simulink model "model"  (R2023b)
settings: Solver=VariableStepAuto  StartTime=0.0  StopTime=10.0  RelTol=1e-3
undefined symbols (not defined in the file): DiscIntNeverNeededParam, fd74c4e2, magnitude, Newton, Raphson
libraries: simulink x102, slpidlib x35
(part 1 of 5)
settings Model: Creator=ojiken  LastModifiedBy=ojiken

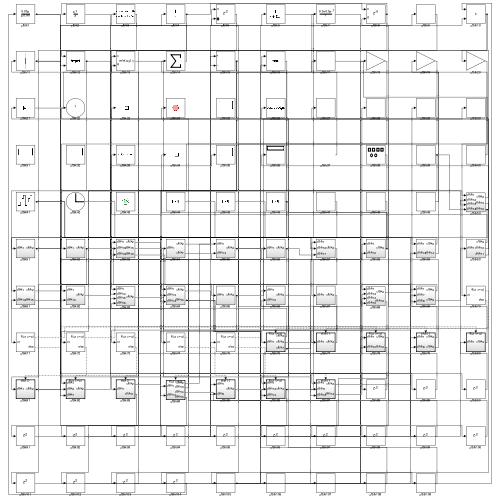
[thumbnail: Simulink's stored preview of the top-level diagram]
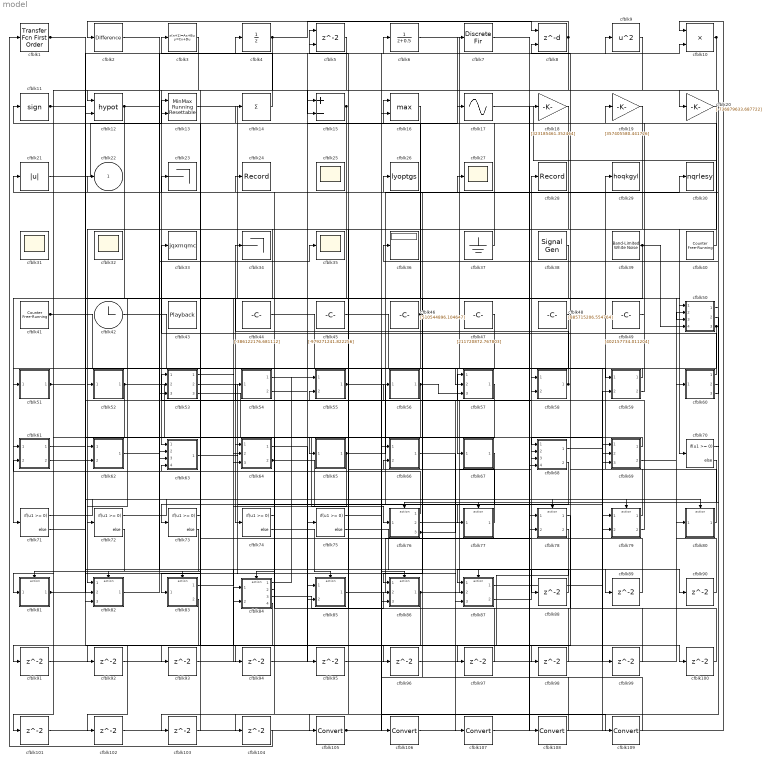
== system model ==
  cfblk1 : simulink/Discrete/Transfer Fcn First Order  PoleZ=0.95  ICPrevOutput=0.0  DoSatur=off
  cfblk10 : Product  Inputs=**
  cfblk{88..104} (17 alike) : Delay  SampleTime=1
  cfblk{105..109} (5 alike) : DataTypeConversion  SaturateOnIntegerOverflow=off  RndMeth=Floor
  cfblk11 : Signum
  cfblk12 : Math  Operator=hypot
  cfblk13 : simulink/Math Operations/MinMax Running Resettable  Function=min  vinit=0.0
  cfblk14 : Sum  Inputs=+
  cfblk15 : Sum  Inputs=+-
  cfblk16 : MinMax  Function=max  Inputs=2
  cfblk17 : Sin  TimeSource=Use external signal  SampleTime=0
  cfblk18 : Gain  Gain=[323185461.352464]
  cfblk19 : Gain  Gain=[357405580.441726]
  cfblk2 : simulink/Discrete/Difference  ICPrevInput=0.0  OutMin=[]  OutMax=[]  OutDataTypeStr=Inherit: Inherit via back propagation  OutDataType=fixdt(1, 16)  OutScaling=2^-10  DoSatur=off
  cfblk20 : Gain  Gain=[-736879633.687722]
  cfblk21 : Abs  SaturateOnIntegerOverflow=off
  cfblk23 : Terminator
  cfblk24 : Record  FileSettingsInternal="{\"entries\":[{\"content\":{\"excelSettings\":{\"content\":{},\"type\":\"Streamout.ExcelSettings\"}},\"type\":\"Streamout.FileSettingStorage\",\"uuid\":\"\"}],\"packageUris\":[\"http:\\/\\/schema.mathworks.com\\/mf0\\/streamout_blocks\\/R2020a\"],\"version\":\"1.0\"}"  SignalsInternal="{\"entries\":[{\"content\":{},\"type\":\"RecordBlkView.InputSignals\",\"uuid\":\"\"}],\"packageUris\":[\"http:\\/\\/schema.mathworks.com\\/mf0\\/streamout_blocks\\/R2020a\"],\"version\":\"1.0\"}"  VisualizationBindings="{\"sparklinesplugin\":{\"info\":[{\"bindingParametersList\":[],\"subplotID\":1}]}}"
  cfblk{25,27,31..32,35} (5 alike) : Scope
      cfblk25 settings: Floating=on
      cfblk31 settings: Floating=on
      cfblk32 settings: Floating=on
  cfblk26 : ToWorkspace  VariableName=lyoptgs  SaveFormat=Timeseries  SampleTime=-1
  cfblk28 : Record  FileSettingsInternal="{\"entries\":[{\"content\":{\"excelSettings\":{\"content\":{},\"type\":\"Streamout.ExcelSettings\"}},\"type\":\"Streamout.FileSettingStorage\",\"uuid\":\"\"}],\"packageUris\":[\"http:\\/\\/schema.mathworks.com\\/mf0\\/streamout_blocks\\/R2020a\"],\"version\":\"1.0\"}"  SignalsInternal="{\"entries\":[{\"content\":{},\"type\":\"RecordBlkView.InputSignals\",\"uuid\":\"\"}],\"packageUris\":[\"http:\\/\\/schema.mathworks.com\\/mf0\\/streamout_blocks\\/R2020a\"],\"version\":\"1.0\"}"  VisualizationBindings="{\"sparklinesplugin\":{\"info\":[{\"bindingParametersList\":[],\"subplotID\":1}]}}"
  cfblk29 : ToWorkspace  VariableName=hoqkgyl  SaveFormat=Timeseries  SampleTime=-1
  cfblk3 : DiscreteStateSpace
  cfblk30 : ToWorkspace  VariableName=nqrlesy  SaveFormat=Timeseries  SampleTime=-1
  cfblk33 : ToWorkspace  VariableName=jqxmqmc  SaveFormat=Timeseries  SampleTime=-1
  cfblk34 : Terminator
  cfblk36 : Display
  cfblk37 : Ground
  cfblk38 : SignalGenerator  Amplitude=[-773767244.573252]  Units=rad/sec
  cfblk39 : simulink/Sources/Band-Limited White Noise  Cov=[9388450366.311230]  Ts=0.1  seed=[6338139783.000000]
  cfblk4 : UnitDelay  HasFrameUpgradeWarning=on
  cfblk40 : simulink/Sources/Counter Free-Running  NumBits=[55.000000]  tsamp=-1
  cfblk41 : simulink/Sources/Counter Free-Running  NumBits=[4.000000]  tsamp=-1
  cfblk42 : Clock
  cfblk43 : Playback  NumPorts=0  PartName=fd74c4e2-0fad-4813-8d20-90b65e462531
  cfblk44 : Constant  Value=[-386122176.681112]  SampleTime=1
  cfblk45 : Constant  Value=[-979271241.822256]  SampleTime=1
  cfblk46 : Constant  Value=[510544896.104647]  SampleTime=1
  cfblk47 : Constant  Value=[211720872.767803]  SampleTime=1
  cfblk48 : Constant  Value=[885715206.554764]  SampleTime=1
  cfblk49 : Constant  Value=[402157734.011204]  SampleTime=1
  cfblk5 : Delay  ShowEnablePort=on  SampleTime=1
      settings: InputPortMap=u0,e6
  cfblk50 : Subsystem
  cfblk51 : Subsystem
  cfblk52 : Subsystem
  cfblk53 : Subsystem
  cfblk54 : Subsystem
  cfblk55 : Subsystem
  cfblk56 : Subsystem
  cfblk57 : Subsystem
  cfblk58 : Subsystem
  cfblk59 : Subsystem
  cfblk6 : DiscreteTransferFcn  SampleTime=1
  cfblk60 : Subsystem
  cfblk61 : Subsystem
  cfblk62 : Subsystem
  cfblk63 : Subsystem
  cfblk64 : Subsystem
  cfblk65 : Subsystem
  cfblk66 : Subsystem
  cfblk67 : Subsystem
  cfblk68 : Subsystem
  cfblk69 : Subsystem
  cfblk7 : DiscreteFir  SampleTime=1
  cfblk{70..75} (6 alike) : If  IfExpression=u1 >= 0  SampleTime=1
  cfblk76 : Subsystem  TreatAsAtomicUnit=on
  cfblk77 : Subsystem  TreatAsAtomicUnit=on
  cfblk78 : Subsystem  TreatAsAtomicUnit=on
  cfblk79 : Subsystem  TreatAsAtomicUnit=on
  cfblk8 : Delay  DelayLengthSource=Input port  SampleTime=1
      settings: InputPortMap=u0,p1
  cfblk80 : Subsystem  TreatAsAtomicUnit=on
  cfblk81 : Subsystem  TreatAsAtomicUnit=on
  cfblk82 : Subsystem  TreatAsAtomicUnit=on
  cfblk83 : Subsystem  TreatAsAtomicUnit=on
  cfblk84 : Subsystem  TreatAsAtomicUnit=on
  cfblk85 : Subsystem  TreatAsAtomicUnit=on
  cfblk86 : Subsystem  TreatAsAtomicUnit=on
  cfblk87 : Subsystem  TreatAsAtomicUnit=on
  cfblk9 : Math  Operator=square
  cfblk22 : Outport
  wires:
  cfblk15/1 -> cfblk72/1, cfblk64/3(cfblk14), cfblk93/1
  cfblk84/1(cfblk2) -> cfblk55/1(cfblk1)
  cfblk3/1 -> cfblk63/1(cfblk1)
  cfblk80/1(cfblk2) -> cfblk29/1
  cfblk65/1(cfblk2) -> cfblk30/1, cfblk84/2(cfblk12)
  cfblk17/1 -> cfblk70/1
  cfblk12/1 -> cfblk82/1(cfblk1), cfblk89/1
  cfblk44/1 -> cfblk76/1(cfblk1)
  cfblk39/1 -> cfblk71/1, cfblk50/4(cfblk14)
  cfblk62/1(cfblk2) -> cfblk9/1
  cfblk46/1 -> cfblk11/1, cfblk62/2(cfblk13), cfblk53/2(cfblk13)
  cfblk48/1 -> cfblk82/2(cfblk6)
  cfblk85/1(cfblk2) -> cfblk28/1
  cfblk54/1(cfblk2) -> cfblk6/1
  cfblk84/2(cfblk13) -> cfblk23/1
  cfblk47/1 -> cfblk61/1(cfblk1)
  cfblk63/1(cfblk2) -> cfblk79/2(cfblk8)
  cfblk6/1 -> cfblk59/1(cfblk1)
  cfblk8/1 -> cfblk2/1, cfblk101/1
  cfblk13/1 -> cfblk50/1(cfblk1)
  cfblk40/1 -> cfblk7/1
  cfblk41/1 -> cfblk68/4(cfblk15), cfblk106/1
  cfblk86/1(cfblk2) -> cfblk58/1(cfblk1), cfblk91/1
  cfblk49/1 -> cfblk19/1
  cfblk51/1(cfblk2) -> cfblk57/2(cfblk16), cfblk88/1
  cfblk53/2(cfblk15) -> cfblk87/2(cfblk11)
  cfblk55/1(cfblk2) -> cfblk87/3(cfblk12), cfblk10/2
  cfblk21/1 -> cfblk13/1
  cfblk45/1 -> cfblk67/1(cfblk1)
  cfblk4/1 -> cfblk83/1(cfblk1), cfblk8/1
  cfblk58/1(cfblk2) -> cfblk34/1, cfblk26/1
  cfblk69/1(cfblk2) -> cfblk68/1(cfblk1)
  cfblk82/1(cfblk2) -> cfblk35/1
  cfblk81/1(cfblk2) -> cfblk4/1, cfblk94/1
  cfblk50/1(cfblk2) -> cfblk20/1
  cfblk56/1(cfblk2) -> cfblk57/3(cfblk17), cfblk104/1
  cfblk60/1(cfblk2) -> cfblk33/1
  cfblk57/1(cfblk2) -> cfblk82/3(cfblk7)
  cfblk79/1(cfblk2) -> cfblk21/1
  cfblk14/1 -> cfblk3/1
  cfblk18/1 -> cfblk105/1
  cfblk20/1 -> cfblk52/1(cfblk1)
  cfblk37/1 -> cfblk14/1
  cfblk1/1 -> cfblk63/2(cfblk14), cfblk85/2(cfblk9)
  cfblk16/1 -> cfblk62/1(cfblk1)
  cfblk59/1(cfblk2) -> cfblk51/1(cfblk1)
  cfblk19/1 -> cfblk74/1
  cfblk5/1 -> cfblk12/1
  cfblk52/1(cfblk2) -> cfblk65/1(cfblk1), cfblk81/1(cfblk1)
  cfblk38/1 -> cfblk86/1(cfblk1)
  cfblk68/1(cfblk2) -> cfblk59/2(cfblk13)
  cfblk61/1(cfblk2) -> cfblk56/1(cfblk1)
  cfblk87/1(cfblk2) -> cfblk69/2(cfblk7)
  cfblk69/2(cfblk9) -> cfblk60/1(cfblk1)
  cfblk87/2(cfblk13) -> cfblk68/2(cfblk13)
  cfblk60/2(cfblk10) -> cfblk36/1
  cfblk9/1 -> cfblk12/2
  cfblk76/1(cfblk2) -> cfblk61/2(cfblk14)
  cfblk77/1(cfblk2) -> cfblk5/1
  cfblk10/1 -> cfblk15/2, cfblk53/3(cfblk14)
  cfblk11/1 -> cfblk5/2, cfblk50/3(cfblk13)
  cfblk60/3(cfblk11) -> cfblk22/1
  cfblk50/3(cfblk16) -> cfblk27/1, cfblk64/2(cfblk13)
  cfblk42/1 -> cfblk69/3(cfblk8)
  cfblk61/2(cfblk15) -> cfblk57/1(cfblk1)
  cfblk79/2(cfblk9) -> cfblk54/1(cfblk1)
  cfblk54/2(cfblk7) -> cfblk17/1
  cfblk64/2(cfblk15) -> cfblk53/1(cfblk1), cfblk86/3(cfblk14), cfblk100/1
  cfblk2/1 -> cfblk64/1(cfblk1)
  cfblk68/2(cfblk16) -> cfblk73/1
  cfblk76/2(cfblk6) -> cfblk68/3(cfblk14)
  cfblk67/1(cfblk2) -> cfblk77/1(cfblk1)
  cfblk59/2(cfblk14) -> cfblk16/1
  cfblk84/3(cfblk14) -> cfblk86/2(cfblk13)
  cfblk76/3(cfblk7) -> cfblk24/1, cfblk58/2(cfblk10)
  cfblk70/1 -> cfblk76/Action
  cfblk70/2 -> cfblk77/Action
  cfblk71/1 -> cfblk78/Action
  cfblk71/2 -> cfblk79/Action
  cfblk72/1 -> cfblk80/Action
  cfblk72/2 -> cfblk81/Action
  cfblk73/1 -> cfblk82/Action
  cfblk73/2 -> cfblk83/Action
  cfblk74/1 -> cfblk84/Action
  cfblk74/2 -> cfblk85/Action
  cfblk75/1 -> cfblk86/Action
  cfblk75/2 -> cfblk87/Action
  cfblk88/1 -> cfblk87/1(cfblk1)
  cfblk89/1 -> cfblk63/4(cfblk16)
  cfblk83/1(cfblk2) -> cfblk90/1
  cfblk90/1 -> cfblk50/2(cfblk12)
  cfblk91/1 -> cfblk84/1(cfblk1)
  cfblk83/2(cfblk11) -> cfblk92/1
  cfblk92/1 -> cfblk75/1
  cfblk93/1 -> cfblk79/1(cfblk1)
  cfblk94/1 -> cfblk15/1
  cfblk64/1(cfblk2) -> cfblk95/1
  cfblk95/1 -> cfblk78/1(cfblk1)
  cfblk78/1(cfblk2) -> cfblk96/1
  cfblk96/1 -> cfblk80/1(cfblk1)
  cfblk78/2(cfblk10) -> cfblk97/1
  cfblk97/1 -> cfblk85/1(cfblk1)
  cfblk53/1(cfblk2) -> cfblk98/1
  cfblk98/1 -> cfblk55/2(cfblk13)
  cfblk53/3(cfblk16) -> cfblk99/1
  cfblk99/1 -> cfblk63/3(cfblk15)
  cfblk100/1 -> cfblk8/2
  cfblk101/1 -> cfblk10/1
  cfblk84/4(cfblk15) -> cfblk102/1
  cfblk102/1 -> cfblk78/2(cfblk9)
  cfblk50/2(cfblk15) -> cfblk103/1
  cfblk103/1 -> cfblk13/2
  cfblk104/1 -> cfblk1/1
  cfblk105/1 -> cfblk16/2, cfblk109/1
  cfblk106/1 -> cfblk18/1
  cfblk66/1(cfblk2) -> cfblk107/1
  cfblk107/1 -> cfblk69/1(cfblk1)
  cfblk7/1 -> cfblk108/1
  cfblk108/1 -> cfblk66/1(cfblk1)
  cfblk109/1 -> cfblk66/2(cfblk12)

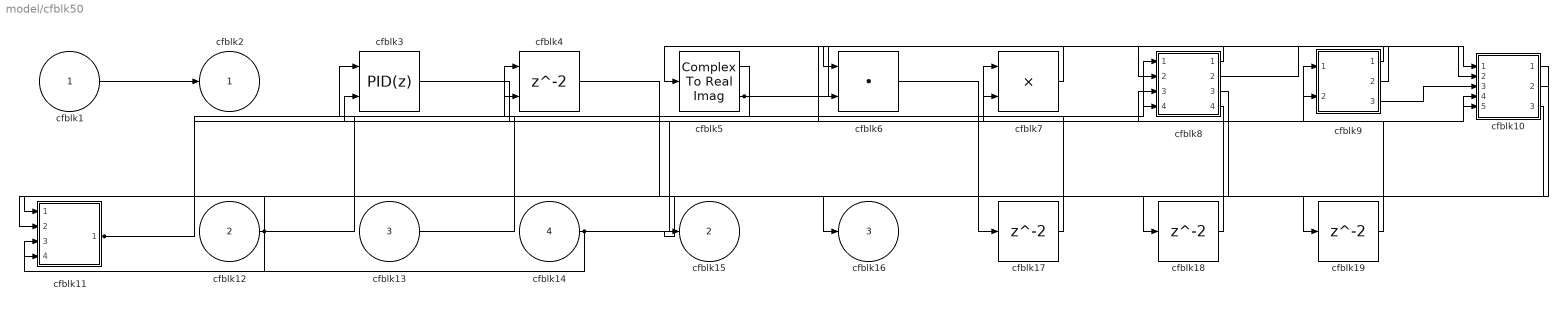
== system model/cfblk50 ==
  cfblk1 : Inport
  cfblk12 : Inport  Port=2
  cfblk13 : Inport  Port=3
  cfblk14 : Inport  Port=4
  cfblk10 : Subsystem
  cfblk11 : Subsystem
  cfblk17 : Delay  SampleTime=1
  cfblk18 : Delay  SampleTime=1
  cfblk19 : Delay  SampleTime=1
  cfblk3 : slpidlib/PID Controller (2DOF)  Controller=PID  Form=Parallel  TimeDomain=Discrete-time  UseExternalTs=off  SampleTime=1  IntegratorMethod=Forward Euler  FilterMethod=Forward Euler  ControllerParametersSource=internal  P=1  I=1  UseKiTs=off  D=0  N=100  UseFilter=on  b=1  c=1  TunerSelectOption=Transfer Function Based (PID Tuner App)  InitialConditionSource=internal  InitialConditionForIntegrator=0  InitialConditionForFilter=0  DifferentiatorICPrevScaledInput=0  ExternalReset=none  TrackingMode=off  Kt=1  LimitOutput=off  SatLimitsSource=internal  UpperSaturationLimit=inf  LowerSaturationLimit=-inf  LinearizeAsGain=off  AntiWindupMode=none  Kb=1  LimitIntegrator=off  UpperIntegratorSaturationLimit=inf  LowerIntegratorSaturationLimit=-inf  POutMin=[]  POutMax=[]  IOutMin=[]  IOutMax=[]  DOutMin=[]  DOutMax=[]  NOutMin=[]  NOutMax=[]  bOutMin=[]  bOutMax=[]  cOutMin=[]  cOutMax=[]  SumOutMin=[]  SumOutMax=[]  SaturationOutMin=[]  SaturationOutMax=[]  PParamMin=[]  PParamMax=[]  IParamMin=[]  IParamMax=[]  DParamMin=[]  DParamMax=[]  NParamMin=[]  NParamMax=[]  bParamMin=[]  bParamMax=[]  cParamMin=[]  cParamMax=[]  KbParamMin=[]  KbParamMax=[]  KtParamMin=[]  KtParamMax=[]  KbOutMin=[]  KbOutMax=[]  KtOutMin=[]  KtOutMax=[]  IntegratorOutMin=[]  IntegratorOutMax=[]  FilterOutMin=[]  FilterOutMax=[]  SumI1OutMin=[]  SumI1OutMax=[]  SumI2OutMin=[]  SumI2OutMax=[]  SumI3OutMin=[]  SumI3OutMax=[]  SumI4OutMin=[]  SumI4OutMax=[]  SumDOutMin=[]  SumDOutMax=[]  Sum1OutMin=[]  Sum1OutMax=[]  Sum2OutMin=[]  Sum2OutMax=[]  Sum3OutMin=[]  Sum3OutMax=[]  DifferentiatorOutMin=[]  DifferentiatorOutMax=[]  FilterDiffOutCoefMin=[]  FilterDiffOutCoefMax=[]  ReciprocalOutMin=[]  ReciprocalOutMax=[]  SumDenOutMin=[]  SumDenOutMax=[]  SumNumOutMin=[]  SumNumOutMax=[]  DivideOutMin=[]  DivideOutMax=[]  UdiffTsProdOutMin=[]  UdiffTsProdOutMax=[]  NTsProdOutMin=[]  NTsProdOutMax=[]  UintegralTsProdOutMin=[]  UintegralTsProdOutMax=[]  UngainTsProdOutMin=[]  UngainTsProdOutMax=[]  ClampingZeroOutDataTypeStr=Inherit: Inherit via back propagation  ClampingZeroOutMin=[]  ClampingZeroOutMax=[]  FilterDenConstantOutDataTypeStr=Inherit: Inherit via back propagation  FilterDenConstantOutMin=[]  FilterDenConstantOutMax=[]  PCopyOutDataTypeStr=Inherit: Inherit via back propagation  PCopyOutMin=[]  PCopyOutMax=[]  NCopyOutDataTypeStr=Inherit: Inherit via back propagation  NCopyOutMin=[]  NCopyOutMax=[]  IntegratorContinuousStateAttributes=''  IntegratorStateMustResolveToSignalObject=off  IntegratorRTWStateStorageClass=Auto  FilterContinuousStateAttributes=''  FilterStateMustResolveToSignalObject=off  FilterRTWStateStorageClass=Auto  ParallelPVariant=InternalParameters  IdealPVariant=Disabled  IVariant=InternalParameters  DVariant=InternalParameters  bVariant=InternalParameters  cVariant=InternalParameters  IntegratorVariant=Discrete  SatVariant=Disabled  AWVariant=Passthrough  PCopyVariant=Disabled  TRVariant=Disabled  FdbkBlocksVariant=Forward  IdealPFdbkVariant=Disabled  SatFdbkVariant=Disabled  DerivativeFilterVariant=ForwardEulerFilter  NVariant=InternalParameters  NCopyVariant=Disabled  FilterICVariant=InternalICsFilter  IntegratorICVariant=InternalICs  ExternalResetVariant=Disabled  TRSumVariant=Passthrough  SumFdbkVariant=Disabled  SumVariant=Sum_PID  TsampFilterVariant=InternalTs  TsampNgainVariant=Passthrough  TsampIntegralVariant=Disabled_SignalSpec  ExternalSaturationOutDataTypeStr=Inherit: Same as second input
      settings: LibrarySourceBlock=simulink/Discrete/Discrete PID Controller (2DOF)
  cfblk4 : Delay  ShowEnablePort=on  SampleTime=1
      settings: InputPortMap=u0,e6
  cfblk5 : ComplexToRealImag
  cfblk6 : DotProduct  OutDataTypeStr=Inherit: Inherit via internal rule
  cfblk7 : Product  Inputs=**
  cfblk8 : Subsystem
  cfblk9 : Subsystem
  cfblk2 : Outport
  cfblk15 : Outport  Port=2
  cfblk16 : Outport  Port=3
  wires:
  cfblk3/1 -> cfblk9/1(cfblk1)
  cfblk1/1 -> cfblk2/1
  cfblk12/1 -> cfblk11/1(cfblk1), cfblk7/2, cfblk8/4(cfblk11), cfblk11/4(cfblk15)
  cfblk11/1(cfblk2) -> cfblk4/1, cfblk10/4(cfblk11)
  cfblk5/1 -> cfblk4/2
  cfblk5/2 -> cfblk10/1(cfblk1), cfblk10/5(cfblk12)
  cfblk8/1(cfblk2) -> cfblk5/1
  cfblk7/1 -> cfblk6/1
  cfblk13/1 -> cfblk8/1(cfblk1)
  cfblk14/1 -> cfblk9/2(cfblk9), cfblk11/3(cfblk14)
  cfblk8/2(cfblk12) -> cfblk10/2(cfblk9)
  cfblk10/1(cfblk2) -> cfblk15/1
  cfblk9/1(cfblk2) -> cfblk6/2
  cfblk9/2(cfblk10) -> cfblk8/2(cfblk9)
  cfblk9/3(cfblk11) -> cfblk10/3(cfblk10)
  cfblk8/3(cfblk13) -> cfblk11/2(cfblk13)
  cfblk8/4(cfblk14) -> cfblk7/1
  cfblk10/2(cfblk13) -> cfblk16/1
  cfblk6/1 -> cfblk17/1
  cfblk17/1 -> cfblk3/1
  cfblk4/1 -> cfblk18/1
  cfblk18/1 -> cfblk3/2
  cfblk10/3(cfblk14) -> cfblk19/1
  cfblk19/1 -> cfblk8/3(cfblk10)

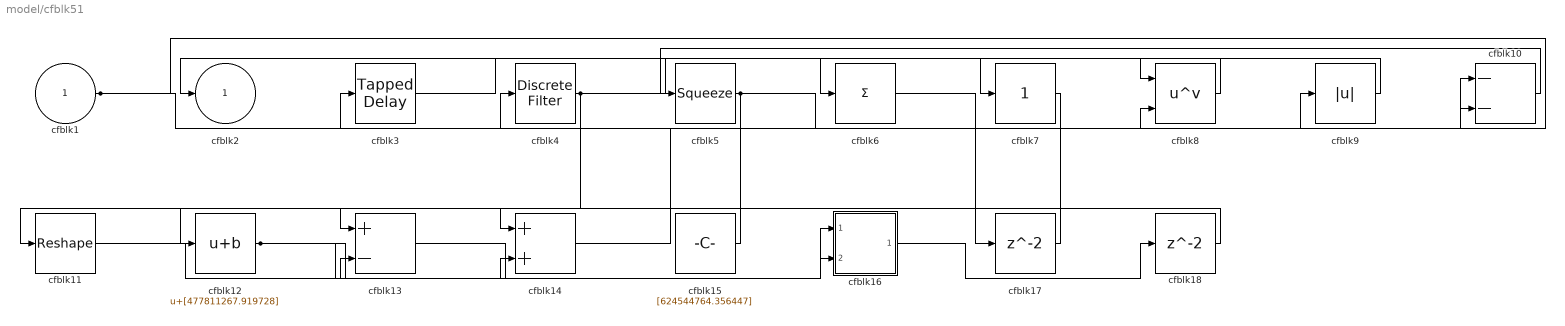
== system model/cfblk51 ==
  cfblk1 : Inport
  cfblk10 : Sum  Inputs=--
  cfblk11 : Reshape
  cfblk12 : Bias  Bias=[477811267.919728]  SaturateOnIntegerOverflow=off
  cfblk13 : Sum  Inputs=+-
  cfblk14 : Sum
  cfblk15 : Constant  Value=[624544764.356447]  SampleTime=1
  cfblk16 : Subsystem
  cfblk17 : Delay  SampleTime=1
  cfblk18 : Delay  SampleTime=1
  cfblk3 : simulink/Discrete/Tapped Delay  vinit=0.0  samptime=-1  NumDelays=1  DelayOrder=Oldest  includeCurrent=off
  cfblk4 : DiscreteFilter  SampleTime=1
  cfblk5 : Squeeze
  cfblk6 : Sum  Inputs=+
  cfblk7 : simulink/Math Operations/Slider Gain  gain=1  low=0  high=2
  cfblk8 : Math  Operator=pow
  cfblk9 : Abs  SaturateOnIntegerOverflow=off
  cfblk2 : Outport
  wires:
  cfblk7/1 -> cfblk11/1
  cfblk4/1 -> cfblk7/1, cfblk12/1
  cfblk15/1 -> cfblk4/1
  cfblk12/1 -> cfblk16/1(cfblk1), cfblk14/2
  cfblk10/1 -> cfblk5/1
  cfblk3/1 -> cfblk6/1
  cfblk11/1 -> cfblk13/2
  cfblk14/1 -> cfblk9/1
  cfblk8/1 -> cfblk2/1
  cfblk5/1 -> cfblk14/1, cfblk8/2
  cfblk9/1 -> cfblk8/1
  cfblk1/1 -> cfblk10/1, cfblk10/2
  cfblk13/1 -> cfblk16/2(cfblk11)
  cfblk6/1 -> cfblk17/1
  cfblk17/1 -> cfblk3/1
  cfblk16/1(cfblk2) -> cfblk18/1
  cfblk18/1 -> cfblk13/1

== system model/cfblk52 ==
  cfblk1 : Inport
  cfblk10 : Subsystem
  cfblk11 : Subsystem
  cfblk{12..17} (6 alike) : Delay  SampleTime=1
  cfblk3 : DiscreteStateSpace
  cfblk4 : Delay  DelayLengthSource=Input port  SampleTime=1
      settings: InputPortMap=u0,p1
  cfblk5 : Sqrt
  cfblk6 : Abs  SaturateOnIntegerOverflow=off
  cfblk7 : Subsystem
  cfblk8 : Subsystem
  cfblk9 : Subsystem
  cfblk2 : Outport
  wires:
  cfblk3/1 -> cfblk13/1, cfblk14/1
  cfblk1/1 -> cfblk8/2(cfblk6)
  cfblk7/1(cfblk2) -> cfblk9/1(cfblk1)
  cfblk5/1 -> cfblk2/1, cfblk15/1
  cfblk11/2(cfblk15) -> cfblk3/1
  cfblk7/2(cfblk12) -> cfblk10/1(cfblk1), cfblk11/2(cfblk13)
  cfblk9/1(cfblk2) -> cfblk11/1(cfblk1)
  cfblk4/1 -> cfblk7/1(cfblk1)
  cfblk11/3(cfblk16) -> cfblk5/1, cfblk16/1
  cfblk8/1(cfblk2) -> cfblk4/2, cfblk6/1
  cfblk6/1 -> cfblk10/2(cfblk6), cfblk11/3(cfblk14), cfblk10/3(cfblk7)
  cfblk11/1(cfblk2) -> cfblk12/1
  cfblk12/1 -> cfblk4/1
  cfblk13/1 -> cfblk8/1(cfblk1)
  cfblk14/1 -> cfblk9/2(cfblk7)
  cfblk15/1 -> cfblk8/3(cfblk7)
  cfblk16/1 -> cfblk8/4(cfblk8)
  cfblk10/1(cfblk2) -> cfblk17/1
  cfblk17/1 -> cfblk7/2(cfblk11)

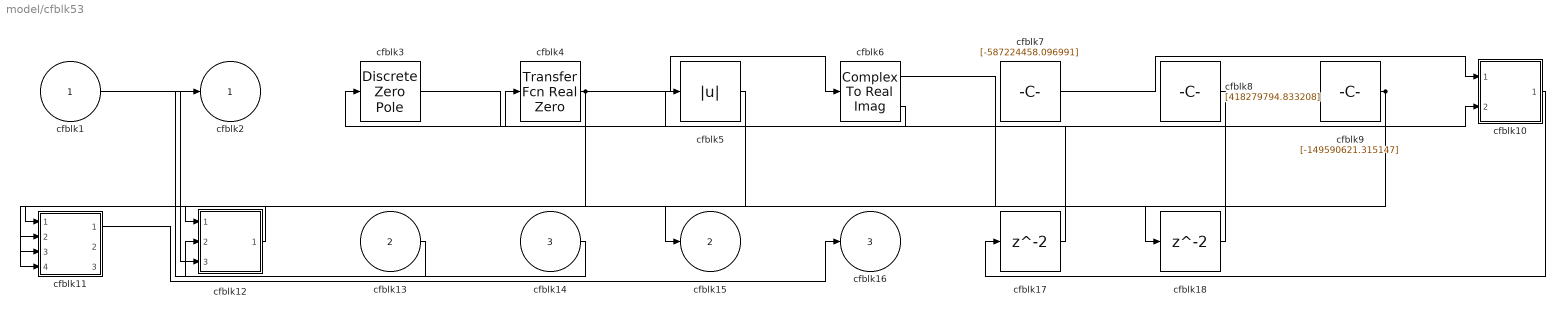
== system model/cfblk53 ==
  cfblk1 : Inport
  cfblk13 : Inport  Port=2
  cfblk14 : Inport  Port=3
  cfblk10 : Subsystem
  cfblk11 : Subsystem
  cfblk12 : Subsystem
  cfblk17 : Delay  SampleTime=1
  cfblk18 : Delay  SampleTime=1
  cfblk3 : DiscreteZeroPole  Poles=[0 0.5]  Gain=1
  cfblk4 : simulink/Discrete/Transfer Fcn Real Zero  ZeroZ=0.75  ICPrevInput=0.0  DoSatur=off
  cfblk5 : Abs  SaturateOnIntegerOverflow=off
  cfblk6 : ComplexToRealImag
  cfblk7 : Constant  Value=[-587224458.096991]  SampleTime=1
  cfblk8 : Constant  Value=[418279794.833208]  SampleTime=1
  cfblk9 : Constant  Value=[-149590621.315147]  SampleTime=1
  cfblk2 : Outport
  cfblk15 : Outport  Port=2
  cfblk16 : Outport  Port=3
  wires:
  cfblk9/1 -> cfblk12/1(cfblk1), cfblk11/3(cfblk8)
  cfblk14/1 -> cfblk2/1
  cfblk7/1 -> cfblk10/1(cfblk1)
  cfblk4/1 -> cfblk6/1, cfblk11/4(cfblk9)
  cfblk6/2 -> cfblk5/1
  cfblk8/1 -> cfblk15/1
  cfblk11/1(cfblk2) -> cfblk16/1
  cfblk3/1 -> cfblk10/2(cfblk10)
  cfblk13/1 -> cfblk12/2(cfblk13)
  cfblk1/1 -> cfblk12/3(cfblk14)
  cfblk12/1(cfblk2) -> cfblk11/1(cfblk1)
  cfblk5/1 -> cfblk11/2(cfblk7)
  cfblk10/1(cfblk2) -> cfblk17/1
  cfblk17/1 -> cfblk3/1
  cfblk6/1 -> cfblk18/1
  cfblk18/1 -> cfblk4/1

== system model/cfblk54 ==
  cfblk1 : Inport
  cfblk{4,8..10} (4 alike) : Delay  SampleTime=1
  cfblk3 : Delay  DelayLengthSource=Input port  SampleTime=1
      settings: InputPortMap=u0,p1
  cfblk5 : MinMax  Inputs=3
  cfblk6 : Gain  Gain=[-108671966.700826]
  cfblk2 : Outport
  cfblk7 : Outport  Port=2
  wires:
  cfblk1/1 -> cfblk2/1
  cfblk6/1 -> cfblk8/1, cfblk9/1
  cfblk5/1 -> cfblk6/1
  cfblk4/1 -> cfblk7/1, cfblk5/2, cfblk10/1
  cfblk3/1 -> cfblk4/1, cfblk5/3
  cfblk8/1 -> cfblk5/1
  cfblk9/1 -> cfblk3/1
  cfblk10/1 -> cfblk3/2

== system model/cfblk55 ==
  cfblk1 : Inport
  cfblk13 : Inport  Port=2
  cfblk10 : Subsystem
  cfblk11 : Subsystem
  cfblk12 : Subsystem
  cfblk{14..17} (4 alike) : Delay  SampleTime=1
  cfblk3 : slpidlib/PID Controller (2DOF)  Controller=PID  Form=Parallel  TimeDomain=Discrete-time  UseExternalTs=off  SampleTime=1  IntegratorMethod=Forward Euler  FilterMethod=Forward Euler  ControllerParametersSource=internal  P=1  I=1  UseKiTs=off  D=0  N=100  UseFilter=on  b=1  c=1  TunerSelectOption=Transfer Function Based (PID Tuner App)  InitialConditionSource=internal  InitialConditionForIntegrator=0  InitialConditionForFilter=0  DifferentiatorICPrevScaledInput=0  ExternalReset=none  TrackingMode=off  Kt=1  LimitOutput=off  SatLimitsSource=internal  UpperSaturationLimit=inf  LowerSaturationLimit=-inf  LinearizeAsGain=off  AntiWindupMode=none  Kb=1  LimitIntegrator=off  UpperIntegratorSaturationLimit=inf  LowerIntegratorSaturationLimit=-inf  POutMin=[]  POutMax=[]  IOutMin=[]  IOutMax=[]  DOutMin=[]  DOutMax=[]  NOutMin=[]  NOutMax=[]  bOutMin=[]  bOutMax=[]  cOutMin=[]  cOutMax=[]  SumOutMin=[]  SumOutMax=[]  SaturationOutMin=[]  SaturationOutMax=[]  PParamMin=[]  PParamMax=[]  IParamMin=[]  IParamMax=[]  DParamMin=[]  DParamMax=[]  NParamMin=[]  NParamMax=[]  bParamMin=[]  bParamMax=[]  cParamMin=[]  cParamMax=[]  KbParamMin=[]  KbParamMax=[]  KtParamMin=[]  KtParamMax=[]  KbOutMin=[]  KbOutMax=[]  KtOutMin=[]  KtOutMax=[]  IntegratorOutMin=[]  IntegratorOutMax=[]  FilterOutMin=[]  FilterOutMax=[]  SumI1OutMin=[]  SumI1OutMax=[]  SumI2OutMin=[]  SumI2OutMax=[]  SumI3OutMin=[]  SumI3OutMax=[]  SumI4OutMin=[]  SumI4OutMax=[]  SumDOutMin=[]  SumDOutMax=[]  Sum1OutMin=[]  Sum1OutMax=[]  Sum2OutMin=[]  Sum2OutMax=[]  Sum3OutMin=[]  Sum3OutMax=[]  DifferentiatorOutMin=[]  DifferentiatorOutMax=[]  FilterDiffOutCoefMin=[]  FilterDiffOutCoefMax=[]  ReciprocalOutMin=[]  ReciprocalOutMax=[]  SumDenOutMin=[]  SumDenOutMax=[]  SumNumOutMin=[]  SumNumOutMax=[]  DivideOutMin=[]  DivideOutMax=[]  UdiffTsProdOutMin=[]  UdiffTsProdOutMax=[]  NTsProdOutMin=[]  NTsProdOutMax=[]  UintegralTsProdOutMin=[]  UintegralTsProdOutMax=[]  UngainTsProdOutMin=[]  UngainTsProdOutMax=[]  ClampingZeroOutDataTypeStr=Inherit: Inherit via back propagation  ClampingZeroOutMin=[]  ClampingZeroOutMax=[]  FilterDenConstantOutDataTypeStr=Inherit: Inherit via back propagation  FilterDenConstantOutMin=[]  FilterDenConstantOutMax=[]  PCopyOutDataTypeStr=Inherit: Inherit via back propagation  PCopyOutMin=[]  PCopyOutMax=[]  NCopyOutDataTypeStr=Inherit: Inherit via back propagation  NCopyOutMin=[]  NCopyOutMax=[]  IntegratorContinuousStateAttributes=''  IntegratorStateMustResolveToSignalObject=off  IntegratorRTWStateStorageClass=Auto  FilterContinuousStateAttributes=''  FilterStateMustResolveToSignalObject=off  FilterRTWStateStorageClass=Auto  ParallelPVariant=InternalParameters  IdealPVariant=Disabled  IVariant=InternalParameters  DVariant=InternalParameters  bVariant=InternalParameters  cVariant=InternalParameters  IntegratorVariant=Discrete  SatVariant=Disabled  AWVariant=Passthrough  PCopyVariant=Disabled  TRVariant=Disabled  FdbkBlocksVariant=Forward  IdealPFdbkVariant=Disabled  SatFdbkVariant=Disabled  DerivativeFilterVariant=ForwardEulerFilter  NVariant=InternalParameters  NCopyVariant=Disabled  FilterICVariant=InternalICsFilter  IntegratorICVariant=InternalICs  ExternalResetVariant=Disabled  TRSumVariant=Passthrough  SumFdbkVariant=Disabled  SumVariant=Sum_PID  TsampFilterVariant=InternalTs  TsampNgainVariant=Passthrough  TsampIntegralVariant=Disabled_SignalSpec  ExternalSaturationOutDataTypeStr=Inherit: Same as second input
      settings: LibrarySourceBlock=simulink/Discrete/Discrete PID Controller (2DOF)
  cfblk4 : slpidlib/PID Controller (2DOF)  Controller=PID  Form=Parallel  TimeDomain=Discrete-time  UseExternalTs=off  SampleTime=1  IntegratorMethod=Forward Euler  FilterMethod=Forward Euler  ControllerParametersSource=internal  P=1  I=1  UseKiTs=off  D=0  N=100  UseFilter=on  b=1  c=1  TunerSelectOption=Transfer Function Based (PID Tuner App)  InitialConditionSource=internal  InitialConditionForIntegrator=0  InitialConditionForFilter=0  DifferentiatorICPrevScaledInput=0  ExternalReset=none  TrackingMode=off  Kt=1  LimitOutput=off  SatLimitsSource=internal  UpperSaturationLimit=inf  LowerSaturationLimit=-inf  LinearizeAsGain=off  AntiWindupMode=none  Kb=1  LimitIntegrator=off  UpperIntegratorSaturationLimit=inf  LowerIntegratorSaturationLimit=-inf  POutMin=[]  POutMax=[]  IOutMin=[]  IOutMax=[]  DOutMin=[]  DOutMax=[]  NOutMin=[]  NOutMax=[]  bOutMin=[]  bOutMax=[]  cOutMin=[]  cOutMax=[]  SumOutMin=[]  SumOutMax=[]  SaturationOutMin=[]  SaturationOutMax=[]  PParamMin=[]  PParamMax=[]  IParamMin=[]  IParamMax=[]  DParamMin=[]  DParamMax=[]  NParamMin=[]  NParamMax=[]  bParamMin=[]  bParamMax=[]  cParamMin=[]  cParamMax=[]  KbParamMin=[]  KbParamMax=[]  KtParamMin=[]  KtParamMax=[]  KbOutMin=[]  KbOutMax=[]  KtOutMin=[]  KtOutMax=[]  IntegratorOutMin=[]  IntegratorOutMax=[]  FilterOutMin=[]  FilterOutMax=[]  SumI1OutMin=[]  SumI1OutMax=[]  SumI2OutMin=[]  SumI2OutMax=[]  SumI3OutMin=[]  SumI3OutMax=[]  SumI4OutMin=[]  SumI4OutMax=[]  SumDOutMin=[]  SumDOutMax=[]  Sum1OutMin=[]  Sum1OutMax=[]  Sum2OutMin=[]  Sum2OutMax=[]  Sum3OutMin=[]  Sum3OutMax=[]  DifferentiatorOutMin=[]  DifferentiatorOutMax=[]  FilterDiffOutCoefMin=[]  FilterDiffOutCoefMax=[]  ReciprocalOutMin=[]  ReciprocalOutMax=[]  SumDenOutMin=[]  SumDenOutMax=[]  SumNumOutMin=[]  SumNumOutMax=[]  DivideOutMin=[]  DivideOutMax=[]  UdiffTsProdOutMin=[]  UdiffTsProdOutMax=[]  NTsProdOutMin=[]  NTsProdOutMax=[]  UintegralTsProdOutMin=[]  UintegralTsProdOutMax=[]  UngainTsProdOutMin=[]  UngainTsProdOutMax=[]  ClampingZeroOutDataTypeStr=Inherit: Inherit via back propagation  ClampingZeroOutMin=[]  ClampingZeroOutMax=[]  FilterDenConstantOutDataTypeStr=Inherit: Inherit via back propagation  FilterDenConstantOutMin=[]  FilterDenConstantOutMax=[]  PCopyOutDataTypeStr=Inherit: Inherit via back propagation  PCopyOutMin=[]  PCopyOutMax=[]  NCopyOutDataTypeStr=Inherit: Inherit via back propagation  NCopyOutMin=[]  NCopyOutMax=[]  IntegratorContinuousStateAttributes=''  IntegratorStateMustResolveToSignalObject=off  IntegratorRTWStateStorageClass=Auto  FilterContinuousStateAttributes=''  FilterStateMustResolveToSignalObject=off  FilterRTWStateStorageClass=Auto  ParallelPVariant=InternalParameters  IdealPVariant=Disabled  IVariant=InternalParameters  DVariant=InternalParameters  bVariant=InternalParameters  cVariant=InternalParameters  IntegratorVariant=Discrete  SatVariant=Disabled  AWVariant=Passthrough  PCopyVariant=Disabled  TRVariant=Disabled  FdbkBlocksVariant=Forward  IdealPFdbkVariant=Disabled  SatFdbkVariant=Disabled  DerivativeFilterVariant=ForwardEulerFilter  NVariant=InternalParameters  NCopyVariant=Disabled  FilterICVariant=InternalICsFilter  IntegratorICVariant=InternalICs  ExternalResetVariant=Disabled  TRSumVariant=Passthrough  SumFdbkVariant=Disabled  SumVariant=Sum_PID  TsampFilterVariant=InternalTs  TsampNgainVariant=Passthrough  TsampIntegralVariant=Disabled_SignalSpec  ExternalSaturationOutDataTypeStr=Inherit: Same as second input
      settings: LibrarySourceBlock=simulink/Discrete/Discrete PID Controller (2DOF)
  cfblk5 : UnaryMinus
  cfblk6 : Math  Operator=pow
  cfblk7 : Bias  Bias=[11384897.367837]  SaturateOnIntegerOverflow=off
  cfblk8 : Trigonometry
  cfblk9 : Constant  Value=[-990748478.835296]  SampleTime=1
  cfblk2 : Outport
  wires:
  cfblk12/2(cfblk12) -> cfblk2/1
  cfblk11/1(cfblk2) -> cfblk3/1
  cfblk1/1 -> cfblk7/1
  cfblk9/1 -> cfblk4/1
  cfblk6/1 -> cfblk4/2, cfblk10/4(cfblk14)
  cfblk10/1(cfblk2) -> cfblk11/2(cfblk9)
  cfblk13/1 -> cfblk10/2(cfblk12), cfblk12/2(cfblk10)
  cfblk11/2(cfblk14) -> cfblk8/1
  cfblk8/1 -> cfblk5/1
  cfblk4/1 -> cfblk10/3(cfblk13), cfblk11/4(cfblk11), cfblk11/6(cfblk13)
  cfblk10/2(cfblk15) -> cfblk12/3(cfblk11), cfblk3/2, cfblk17/1
  cfblk5/1 -> cfblk12/1(cfblk1), cfblk16/1
  cfblk7/1 -> cfblk6/2, cfblk11/3(cfblk10)
  cfblk3/1 -> cfblk14/1
  cfblk14/1 -> cfblk10/1(cfblk1)
  cfblk12/1(cfblk2) -> cfblk15/1
  cfblk15/1 -> cfblk11/1(cfblk1)
  cfblk16/1 -> cfblk11/5(cfblk12)
  cfblk17/1 -> cfblk6/1

== system model/cfblk56 ==
  cfblk1 : Inport
  cfblk10 : Subsystem
  cfblk11 : Delay  SampleTime=1
  cfblk12 : Delay  SampleTime=1
  cfblk3 : slpidlib/PID Controller (2DOF)  Controller=PID  Form=Parallel  TimeDomain=Discrete-time  UseExternalTs=off  SampleTime=1  IntegratorMethod=Forward Euler  FilterMethod=Forward Euler  ControllerParametersSource=internal  P=1  I=1  UseKiTs=off  D=0  N=100  UseFilter=on  b=1  c=1  TunerSelectOption=Transfer Function Based (PID Tuner App)  InitialConditionSource=internal  InitialConditionForIntegrator=0  InitialConditionForFilter=0  DifferentiatorICPrevScaledInput=0  ExternalReset=none  TrackingMode=off  Kt=1  LimitOutput=off  SatLimitsSource=internal  UpperSaturationLimit=inf  LowerSaturationLimit=-inf  LinearizeAsGain=off  AntiWindupMode=none  Kb=1  LimitIntegrator=off  UpperIntegratorSaturationLimit=inf  LowerIntegratorSaturationLimit=-inf  POutMin=[]  POutMax=[]  IOutMin=[]  IOutMax=[]  DOutMin=[]  DOutMax=[]  NOutMin=[]  NOutMax=[]  bOutMin=[]  bOutMax=[]  cOutMin=[]  cOutMax=[]  SumOutMin=[]  SumOutMax=[]  SaturationOutMin=[]  SaturationOutMax=[]  PParamMin=[]  PParamMax=[]  IParamMin=[]  IParamMax=[]  DParamMin=[]  DParamMax=[]  NParamMin=[]  NParamMax=[]  bParamMin=[]  bParamMax=[]  cParamMin=[]  cParamMax=[]  KbParamMin=[]  KbParamMax=[]  KtParamMin=[]  KtParamMax=[]  KbOutMin=[]  KbOutMax=[]  KtOutMin=[]  KtOutMax=[]  IntegratorOutMin=[]  IntegratorOutMax=[]  FilterOutMin=[]  FilterOutMax=[]  SumI1OutMin=[]  SumI1OutMax=[]  SumI2OutMin=[]  SumI2OutMax=[]  SumI3OutMin=[]  SumI3OutMax=[]  SumI4OutMin=[]  SumI4OutMax=[]  SumDOutMin=[]  SumDOutMax=[]  Sum1OutMin=[]  Sum1OutMax=[]  Sum2OutMin=[]  Sum2OutMax=[]  Sum3OutMin=[]  Sum3OutMax=[]  DifferentiatorOutMin=[]  DifferentiatorOutMax=[]  FilterDiffOutCoefMin=[]  FilterDiffOutCoefMax=[]  ReciprocalOutMin=[]  ReciprocalOutMax=[]  SumDenOutMin=[]  SumDenOutMax=[]  SumNumOutMin=[]  SumNumOutMax=[]  DivideOutMin=[]  DivideOutMax=[]  UdiffTsProdOutMin=[]  UdiffTsProdOutMax=[]  NTsProdOutMin=[]  NTsProdOutMax=[]  UintegralTsProdOutMin=[]  UintegralTsProdOutMax=[]  UngainTsProdOutMin=[]  UngainTsProdOutMax=[]  ClampingZeroOutDataTypeStr=Inherit: Inherit via back propagation  ClampingZeroOutMin=[]  ClampingZeroOutMax=[]  FilterDenConstantOutDataTypeStr=Inherit: Inherit via back propagation  FilterDenConstantOutMin=[]  FilterDenConstantOutMax=[]  PCopyOutDataTypeStr=Inherit: Inherit via back propagation  PCopyOutMin=[]  PCopyOutMax=[]  NCopyOutDataTypeStr=Inherit: Inherit via back propagation  NCopyOutMin=[]  NCopyOutMax=[]  IntegratorContinuousStateAttributes=''  IntegratorStateMustResolveToSignalObject=off  IntegratorRTWStateStorageClass=Auto  FilterContinuousStateAttributes=''  FilterStateMustResolveToSignalObject=off  FilterRTWStateStorageClass=Auto  ParallelPVariant=InternalParameters  IdealPVariant=Disabled  IVariant=InternalParameters  DVariant=InternalParameters  bVariant=InternalParameters  cVariant=InternalParameters  IntegratorVariant=Discrete  SatVariant=Disabled  AWVariant=Passthrough  PCopyVariant=Disabled  TRVariant=Disabled  FdbkBlocksVariant=Forward  IdealPFdbkVariant=Disabled  SatFdbkVariant=Disabled  DerivativeFilterVariant=ForwardEulerFilter  NVariant=InternalParameters  NCopyVariant=Disabled  FilterICVariant=InternalICsFilter  IntegratorICVariant=InternalICs  ExternalResetVariant=Disabled  TRSumVariant=Passthrough  SumFdbkVariant=Disabled  SumVariant=Sum_PID  TsampFilterVariant=InternalTs  TsampNgainVariant=Passthrough  TsampIntegralVariant=Disabled_SignalSpec  ExternalSaturationOutDataTypeStr=Inherit: Same as second input
      settings: LibrarySourceBlock=simulink/Discrete/Discrete PID Controller (2DOF)
  cfblk4 : DiscreteFilter  SampleTime=1
  cfblk5 : Gain  Gain=[100548473.523188]
  cfblk6 : simulink/Math Operations/MinMax Running Resettable  Function=min  vinit=0.0
  cfblk7 : Constant  Value=[-755077908.990975]  SampleTime=1
  cfblk8 : Subsystem
  cfblk9 : Subsystem
  cfblk2 : Outport
  wires:
  cfblk9/1(cfblk2) -> cfblk3/1
  cfblk9/2(cfblk8) -> cfblk2/1
  cfblk8/1(cfblk2) -> cfblk4/1
  cfblk7/1 -> cfblk3/2
  cfblk10/1(cfblk2) -> cfblk5/1
  cfblk3/1 -> cfblk8/1(cfblk1)
  cfblk6/1 -> cfblk9/2(cfblk7), cfblk10/2(cfblk7)
  cfblk1/1 -> cfblk6/1
  cfblk4/1 -> cfblk10/1(cfblk1), cfblk10/3(cfblk8)
  cfblk5/1 -> cfblk11/1
  cfblk11/1 -> cfblk9/1(cfblk1)
  cfblk8/2(cfblk9) -> cfblk12/1
  cfblk12/1 -> cfblk6/2

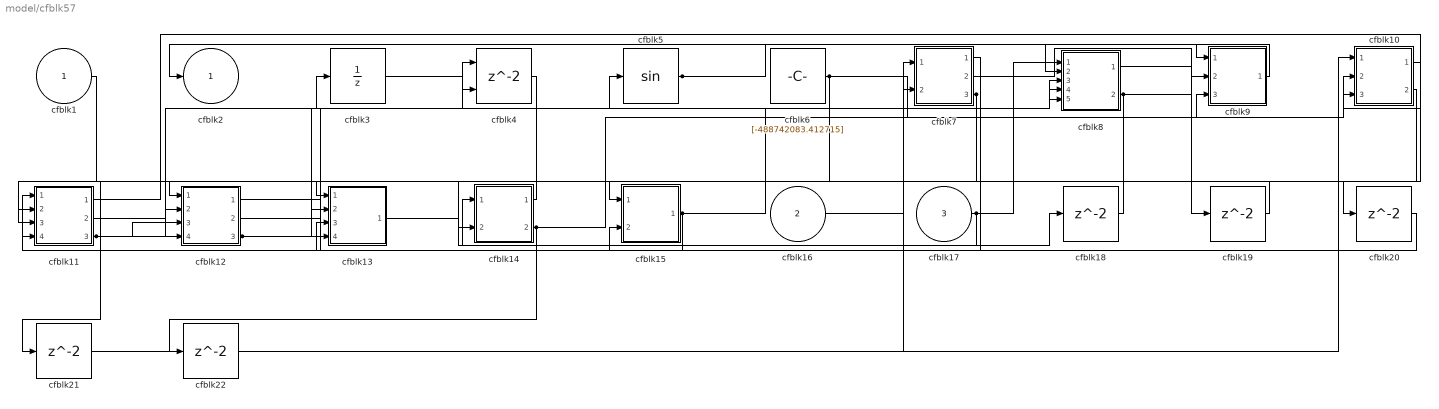
== system model/cfblk57 ==
  cfblk1 : Inport
  cfblk16 : Inport  Port=2
  cfblk17 : Inport  Port=3
  cfblk10 : Subsystem
  cfblk11 : Subsystem
  cfblk12 : Subsystem
  cfblk13 : Subsystem
  cfblk14 : Subsystem
  cfblk15 : Subsystem
  cfblk{18..22} (5 alike) : Delay  SampleTime=1
  cfblk3 : UnitDelay  HasFrameUpgradeWarning=on
  cfblk4 : Delay  ShowEnablePort=on  SampleTime=1
      settings: InputPortMap=u0,e6
  cfblk5 : Trigonometry
  cfblk6 : Constant  Value=[-488742083.412715]  SampleTime=1
  cfblk7 : Subsystem
  cfblk8 : Subsystem
  cfblk9 : Subsystem
  cfblk2 : Outport
  wires:
  cfblk14/1(cfblk2) -> cfblk3/1
  cfblk7/1(cfblk2) -> cfblk11/1(cfblk1)
  cfblk9/1(cfblk2) -> cfblk2/1
  cfblk11/1(cfblk2) -> cfblk10/2(cfblk15)
  cfblk17/1 -> cfblk14/1(cfblk1), cfblk8/1(cfblk1)
  cfblk5/1 -> cfblk9/1(cfblk1), cfblk8/2(cfblk8)
  cfblk12/1(cfblk2) -> cfblk15/1(cfblk1)
  cfblk12/2(cfblk16) -> cfblk15/2(cfblk15)
  cfblk12/3(cfblk17) -> cfblk4/1, cfblk8/4(cfblk10)
  cfblk3/1 -> cfblk4/2
  cfblk10/1(cfblk2) -> cfblk12/2(cfblk13)
  cfblk7/2(cfblk12) -> cfblk9/2(cfblk12)
  cfblk16/1 -> cfblk7/1(cfblk1)
  cfblk6/1 -> cfblk9/3(cfblk13), cfblk12/4(cfblk15)
  cfblk1/1 -> cfblk11/3(cfblk11)
  cfblk8/2(cfblk12) -> cfblk13/4(cfblk13), cfblk20/1
  cfblk7/3(cfblk13) -> cfblk13/1(cfblk1), cfblk14/2(cfblk10)
  cfblk14/2(cfblk11) -> cfblk10/3(cfblk16), cfblk22/1
  cfblk11/2(cfblk13) -> cfblk5/1
  cfblk10/2(cfblk17) -> cfblk13/2(cfblk11)
  cfblk15/1(cfblk2) -> cfblk13/3(cfblk12), cfblk8/3(cfblk9)
  cfblk11/3(cfblk14) -> cfblk12/3(cfblk14), cfblk8/5(cfblk11)
  cfblk13/1(cfblk2) -> cfblk18/1
  cfblk18/1 -> cfblk12/1(cfblk1)
  cfblk8/1(cfblk2) -> cfblk19/1
  cfblk19/1 -> cfblk11/2(cfblk10)
  cfblk20/1 -> cfblk11/4(cfblk12)
  cfblk4/1 -> cfblk21/1
  cfblk21/1 -> cfblk10/1(cfblk1)
  cfblk22/1 -> cfblk7/2(cfblk11)

== system model/cfblk58 ==
  cfblk1 : Inport
  cfblk10 : Inport  Port=2
  cfblk{11..15} (5 alike) : Delay  SampleTime=1
  cfblk3 : Delay  DelayLengthSource=Input port  SampleTime=1
      settings: InputPortMap=u0,p1
  cfblk4 : Gain  Gain=[675508324.106097]
  cfblk5 : Sum  Inputs=+-
  cfblk6 : Sum  Inputs=+
  cfblk7 : Constant  Value=[504559482.739236]  SampleTime=1
  cfblk8 : Subsystem
  cfblk9 : Subsystem
  cfblk2 : Outport
  wires:
  cfblk7/1 -> cfblk4/1
  cfblk5/1 -> cfblk3/1, cfblk15/1
  cfblk4/1 -> cfblk9/1(cfblk1), cfblk8/6(cfblk13)
  cfblk8/1(cfblk2) -> cfblk9/2(cfblk9)
  cfblk6/1 -> cfblk2/1
  cfblk9/1(cfblk2) -> cfblk3/2
  cfblk10/1 -> cfblk9/3(cfblk10)
  cfblk9/2(cfblk11) -> cfblk12/1, cfblk13/1, cfblk14/1
  cfblk8/2(cfblk15) -> cfblk6/1
  cfblk1/1 -> cfblk8/3(cfblk10)
  cfblk8/3(cfblk16) -> cfblk5/1
  cfblk8/4(cfblk17) -> cfblk5/2
  cfblk3/1 -> cfblk11/1
  cfblk11/1 -> cfblk8/1(cfblk1)
  cfblk12/1 -> cfblk8/2(cfblk9)
  cfblk13/1 -> cfblk8/5(cfblk12)
  cfblk14/1 -> cfblk8/7(cfblk14)
  cfblk15/1 -> cfblk8/4(cfblk11)

== system model/cfblk59 ==
  cfblk1 : Inport
  cfblk13 : Inport  Port=2
  cfblk10 : Subsystem
  cfblk11 : Subsystem
  cfblk12 : Subsystem
  cfblk15 : Delay  SampleTime=1
  cfblk16 : Delay  SampleTime=1
  cfblk3 : simulink/Discrete/Transfer Fcn First Order  PoleZ=0.95  ICPrevOutput=0.0  DoSatur=off
  cfblk4 : Abs  SaturateOnIntegerOverflow=off
  cfblk5 : Product  Inputs=**
  cfblk6 : Signum
  cfblk7 : ComplexToMagnitudeAngle
  cfblk8 : Sum  Inputs=|++
  cfblk9 : Constant  Value=[391496658.792457]  SampleTime=1
  cfblk2 : Outport
  cfblk14 : Outport  Port=2
  wires:
  cfblk1/1 -> cfblk8/1
  cfblk5/1 -> cfblk7/1
  cfblk12/1(cfblk2) -> cfblk6/1
  cfblk13/1 -> cfblk10/1(cfblk1), cfblk10/5(cfblk14)
  cfblk11/1(cfblk2) -> cfblk12/2(cfblk8)
  cfblk6/1 -> cfblk10/2(cfblk11)
  cfblk8/1 -> cfblk4/1
  cfblk10/1(cfblk2) -> cfblk3/1
  cfblk11/2(cfblk8) -> cfblk5/2
  cfblk10/2(cfblk16) -> cfblk14/1
  cfblk4/1 -> cfblk11/1(cfblk1), cfblk10/6(cfblk15)
  cfblk9/1 -> cfblk8/2, cfblk10/4(cfblk13)
  cfblk11/3(cfblk9) -> cfblk2/1
  cfblk7/2 -> cfblk10/3(cfblk12)
  cfblk3/1 -> cfblk15/1
  cfblk15/1 -> cfblk12/1(cfblk1)
  cfblk7/1 -> cfblk16/1
  cfblk16/1 -> cfblk5/1

== system model/cfblk60 ==
  cfblk1 : Inport
  cfblk12 : Delay  SampleTime=1
  cfblk13 : Delay  SampleTime=1
  cfblk3 : simulink/Discrete/Transfer Fcn Lead or Lag  PoleZ=0.95  ZeroZ=0.75  ICPrevOutput=0.0  ICPrevInput=0.0  DoSatur=off
  cfblk4 : DiscreteZeroPole  Poles=[0 0.5]  Gain=1
  cfblk5 : MinMax  Function=max  Inputs=3
  cfblk6 : PermuteDimensions
  cfblk7 : Sin  TimeSource=Use external signal  SampleTime=0
  cfblk8 : Subsystem
  cfblk9 : Subsystem
  cfblk2 : Outport
  cfblk10 : Outport  Port=2
  cfblk11 : Outport  Port=3
  wires:
  cfblk9/1(cfblk2) -> cfblk7/1
  cfblk5/1 -> cfblk11/1, cfblk9/2(cfblk10)
  cfblk8/1(cfblk2) -> cfblk10/1
  cfblk8/2(cfblk13) -> cfblk4/1
  cfblk3/1 -> cfblk9/1(cfblk1), cfblk6/1
  cfblk1/1 -> cfblk8/2(cfblk9), cfblk8/5(cfblk12)
  cfblk8/3(cfblk14) -> cfblk2/1
  cfblk6/1 -> cfblk8/3(cfblk10), cfblk8/4(cfblk11), cfblk5/3, cfblk9/3(cfblk11), cfblk13/1
  cfblk4/1 -> cfblk5/1, cfblk5/2
  cfblk7/1 -> cfblk12/1
  cfblk12/1 -> cfblk8/1(cfblk1)
  cfblk13/1 -> cfblk3/1

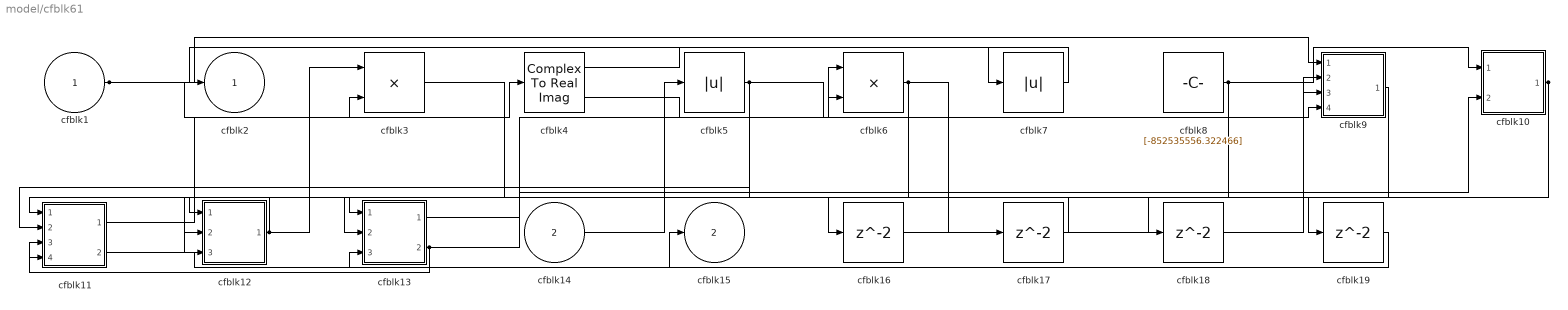
== system model/cfblk61 ==
  cfblk1 : Inport
  cfblk14 : Inport  Port=2
  cfblk10 : Subsystem
  cfblk11 : Subsystem
  cfblk12 : Subsystem
  cfblk13 : Subsystem
  cfblk{16..19} (4 alike) : Delay  SampleTime=1
  cfblk3 : Product  Inputs=**
  cfblk4 : ComplexToRealImag
  cfblk5 : Abs  SaturateOnIntegerOverflow=off
  cfblk6 : Product
  cfblk7 : Abs  SaturateOnIntegerOverflow=off
  cfblk8 : Constant  Value=[-852535556.322466]  SampleTime=1
  cfblk9 : Subsystem
  cfblk2 : Outport
  cfblk15 : Outport  Port=2
  wires:
  cfblk12/1(cfblk2) -> cfblk11/1(cfblk1), cfblk3/1
  cfblk5/1 -> cfblk11/2(cfblk10), cfblk9/4(cfblk15), cfblk12/3(cfblk11)
  cfblk4/1 -> cfblk7/1
  cfblk11/1(cfblk2) -> cfblk4/1
  cfblk8/1 -> cfblk10/1(cfblk1), cfblk12/2(cfblk10)
  cfblk11/2(cfblk13) -> cfblk15/1
  cfblk13/1(cfblk2) -> cfblk10/2(cfblk10)
  cfblk1/1 -> cfblk9/1(cfblk1), cfblk3/2
  cfblk13/2(cfblk14) -> cfblk6/1, cfblk11/3(cfblk11), cfblk11/4(cfblk12)
  cfblk4/2 -> cfblk6/2
  cfblk6/1 -> cfblk16/1, cfblk17/1
  cfblk10/1(cfblk2) -> cfblk12/1(cfblk1), cfblk19/1
  cfblk14/1 -> cfblk5/1
  cfblk7/1 -> cfblk2/1
  cfblk9/1(cfblk2) -> cfblk13/1(cfblk1)
  cfblk16/1 -> cfblk9/2(cfblk13)
  cfblk17/1 -> cfblk13/2(cfblk12)
  cfblk3/1 -> cfblk18/1
  cfblk18/1 -> cfblk9/3(cfblk14)
  cfblk19/1 -> cfblk13/3(cfblk13)

== system model/cfblk62 ==
  cfblk1 : Inport
  cfblk13 : Inport  Port=2
  cfblk10 : Constant  Value=[-832189116.006861]  SampleTime=1
  cfblk11 : Subsystem
  cfblk12 : Subsystem
  cfblk14 : Delay  SampleTime=1
  cfblk3 : simulink/Discrete/Transfer Fcn Lead or Lag  PoleZ=0.95  ZeroZ=0.75  ICPrevOutput=0.0  ICPrevInput=0.0  DoSatur=off
  cfblk4 : simulink/Discrete/Transfer Fcn Real Zero  ZeroZ=0.75  ICPrevInput=0.0  DoSatur=off
  cfblk5 : Trigonometry
  cfblk6 : Reshape
  cfblk7 : Gain  Gain=[373152836.479357]
  cfblk8 : simulink/Math Operations/Slider Gain  gain=1  low=0  high=2
  cfblk9 : Product
  cfblk2 : Outport
  wires:
  cfblk10/1 -> cfblk5/1
  cfblk9/1 -> cfblk2/1
  cfblk12/1(cfblk2) -> cfblk6/1, cfblk9/2
  cfblk5/1 -> cfblk8/1
  cfblk4/1 -> cfblk3/1
  cfblk13/1 -> cfblk7/1
  cfblk1/1 -> cfblk11/1(cfblk1)
  cfblk7/1 -> cfblk12/1(cfblk1), cfblk9/1
  cfblk3/1 -> cfblk12/3(cfblk14)
  cfblk11/1(cfblk2) -> cfblk4/1
  cfblk8/1 -> cfblk12/4(cfblk15)
  cfblk6/1 -> cfblk14/1
  cfblk14/1 -> cfblk12/2(cfblk13)

== system model/cfblk63 ==
  cfblk1 : Inport
  cfblk14 : Inport  Port=2
  cfblk15 : Inport  Port=3
  cfblk16 : Inport  Port=4
  cfblk10 : Sum  Inputs=+
  cfblk11 : Sum  Inputs=|++
  cfblk12 : Squeeze
  cfblk13 : Subsystem
  cfblk17 : Delay  SampleTime=1
  cfblk3 : simulink/Discrete/Transfer Fcn First Order  PoleZ=0.95  ICPrevOutput=0.0  DoSatur=off
  cfblk4 : DiscreteFir  SampleTime=1
  cfblk5 : simulink/Discrete/Transfer Fcn Real Zero  ZeroZ=0.75  ICPrevInput=0.0  DoSatur=off
  cfblk6 : Gain  Gain=[776426309.759099]
  cfblk7 : ComplexToRealImag
  cfblk8 : Sin  TimeSource=Use external signal  SampleTime=0
  cfblk9 : UnaryMinus
  cfblk2 : Outport
  wires:
  cfblk12/1 -> cfblk4/1
  cfblk4/1 -> cfblk7/1
  cfblk14/1 -> cfblk2/1
  cfblk13/1(cfblk2) -> cfblk6/1
  cfblk5/1 -> cfblk10/1
  cfblk15/1 -> cfblk12/1
  cfblk11/1 -> cfblk9/1
  cfblk10/1 -> cfblk8/1
  cfblk16/1 -> cfblk3/1
  cfblk1/1 -> cfblk5/1
  cfblk9/1 -> cfblk13/2(cfblk7)
  cfblk8/1 -> cfblk11/1
  cfblk7/1 -> cfblk13/3(cfblk8)
  cfblk3/1 -> cfblk13/4(cfblk9)
  cfblk7/2 -> cfblk11/2
  cfblk6/1 -> cfblk17/1
  cfblk17/1 -> cfblk13/1(cfblk1)

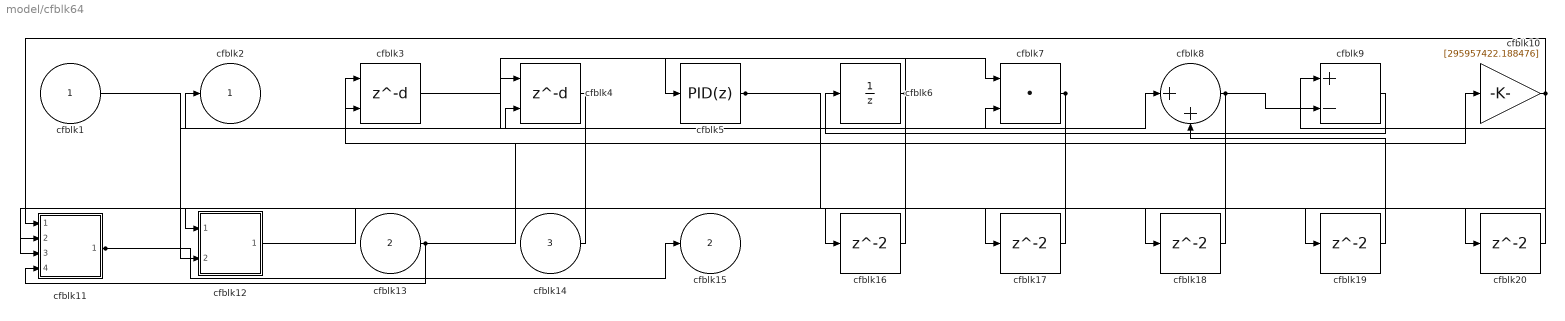
== system model/cfblk64 ==
  cfblk1 : Inport
  cfblk13 : Inport  Port=2
  cfblk14 : Inport  Port=3
  cfblk10 : Gain  Gain=[295957422.188476]
  cfblk11 : Subsystem
  cfblk12 : Subsystem
  cfblk{16..20} (5 alike) : Delay  SampleTime=1
  cfblk3 : Delay  DelayLengthSource=Input port  SampleTime=1
      settings: InputPortMap=u0,p1
  cfblk4 : Delay  DelayLengthSource=Input port  SampleTime=1
      settings: InputPortMap=u0,p1
  cfblk5 : slpidlib/PID Controller  Controller=PID  Form=Parallel  TimeDomain=Discrete-time  UseExternalTs=off  SampleTime=1  IntegratorMethod=Forward Euler  FilterMethod=Forward Euler  ControllerParametersSource=internal  P=1  I=1  UseKiTs=off  D=0  N=100  UseFilter=on  TunerSelectOption=Transfer Function Based (PID Tuner App)  InitialConditionSource=internal  InitialConditionForIntegrator=0  InitialConditionForFilter=0  DifferentiatorICPrevScaledInput=0  ExternalReset=none  TrackingMode=off  Kt=1  LimitOutput=off  SatLimitsSource=internal  UpperSaturationLimit=inf  LowerSaturationLimit=-inf  LinearizeAsGain=off  AntiWindupMode=none  Kb=1  LimitIntegrator=off  UpperIntegratorSaturationLimit=inf  LowerIntegratorSaturationLimit=-inf  POutMin=[]  POutMax=[]  IOutMin=[]  IOutMax=[]  DOutMin=[]  DOutMax=[]  NOutMin=[]  NOutMax=[]  SumOutMin=[]  SumOutMax=[]  SaturationOutMin=[]  SaturationOutMax=[]  PParamMin=[]  PParamMax=[]  IParamMin=[]  IParamMax=[]  DParamMin=[]  DParamMax=[]  NParamMin=[]  NParamMax=[]  KbParamMin=[]  KbParamMax=[]  KtParamMin=[]  KtParamMax=[]  KbOutMin=[]  KbOutMax=[]  KtOutMin=[]  KtOutMax=[]  IntegratorOutMin=[]  IntegratorOutMax=[]  FilterOutMin=[]  FilterOutMax=[]  SumI1OutMin=[]  SumI1OutMax=[]  SumI2OutMin=[]  SumI2OutMax=[]  SumI3OutMin=[]  SumI3OutMax=[]  SumI4OutMin=[]  SumI4OutMax=[]  SumDOutMin=[]  SumDOutMax=[]  DifferentiatorOutMin=[]  DifferentiatorOutMax=[]  FilterDiffOutCoefMin=[]  FilterDiffOutCoefMax=[]  ReciprocalOutMin=[]  ReciprocalOutMax=[]  SumDenOutMin=[]  SumDenOutMax=[]  SumNumOutMin=[]  SumNumOutMax=[]  DivideOutMin=[]  DivideOutMax=[]  UdiffTsProdOutMin=[]  UdiffTsProdOutMax=[]  NTsProdOutMin=[]  NTsProdOutMax=[]  UintegralTsProdOutMin=[]  UintegralTsProdOutMax=[]  UngainTsProdOutMin=[]  UngainTsProdOutMax=[]  ClampingZeroOutDataTypeStr=Inherit: Inherit via back propagation  ClampingZeroOutMin=[]  ClampingZeroOutMax=[]  FilterDenConstantOutDataTypeStr=Inherit: Inherit via back propagation  FilterDenConstantOutMin=[]  FilterDenConstantOutMax=[]  PCopyOutDataTypeStr=Inherit: Inherit via back propagation  PCopyOutMin=[]  PCopyOutMax=[]  NCopyOutDataTypeStr=Inherit: Inherit via back propagation  NCopyOutMin=[]  NCopyOutMax=[]  IntegratorContinuousStateAttributes=''  IntegratorStateMustResolveToSignalObject=off  IntegratorRTWStateStorageClass=Auto  FilterContinuousStateAttributes=''  FilterStateMustResolveToSignalObject=off  FilterRTWStateStorageClass=Auto  ParallelPVariant=InternalParameters  IdealPVariant=Disabled  IVariant=InternalParameters  DVariant=InternalParameters  IntegratorVariant=Discrete  SatVariant=Disabled  AWVariant=Passthrough  PCopyVariant=Disabled  TRVariant=Disabled  FdbkBlocksVariant=Forward  IdealPFdbkVariant=Disabled  SatFdbkVariant=Disabled  DerivativeFilterVariant=ForwardEulerFilter  NVariant=InternalParameters  NCopyVariant=Disabled  FilterICVariant=InternalICsFilter  IntegratorICVariant=InternalICs  ExternalResetVariant=Disabled  TRSumVariant=Passthrough  SumFdbkVariant=Disabled  SumVariant=Sum_PID  TsampFilterVariant=InternalTs  TsampNgainVariant=Passthrough  TsampIntegralVariant=Disabled_SignalSpec  ExternalSaturationOutDataTypeStr=Inherit: Same as second input
      settings: LibrarySourceBlock=simulink/Discrete/Discrete PID Controller
  cfblk6 : UnitDelay  HasFrameUpgradeWarning=on
  cfblk7 : DotProduct  OutDataTypeStr=Inherit: Inherit via internal rule
  cfblk8 : Sum  Inputs=|++
  cfblk9 : Sum  Inputs=+-
  cfblk2 : Outport
  cfblk15 : Outport  Port=2
  wires:
  cfblk7/1 -> cfblk11/2(cfblk12), cfblk11/3(cfblk13), cfblk16/1
  cfblk9/1 -> cfblk6/1
  cfblk4/1 -> cfblk3/1
  cfblk13/1 -> cfblk10/1, cfblk11/4(cfblk14)
  cfblk6/1 -> cfblk5/1, cfblk12/1(cfblk1)
  cfblk11/1(cfblk2) -> cfblk15/1, cfblk8/1
  cfblk3/1 -> cfblk7/1
  cfblk14/1 -> cfblk2/1
  cfblk8/1 -> cfblk9/2, cfblk17/1
  cfblk1/1 -> cfblk4/2
  cfblk5/1 -> cfblk18/1, cfblk19/1
  cfblk10/1 -> cfblk11/1(cfblk1), cfblk12/2(cfblk7)
  cfblk16/1 -> cfblk4/1
  cfblk17/1 -> cfblk7/2
  cfblk18/1 -> cfblk3/2
  cfblk19/1 -> cfblk8/2
  cfblk12/1(cfblk2) -> cfblk20/1
  cfblk20/1 -> cfblk9/1

== system model/cfblk65 ==
  cfblk1 : Inport
  cfblk10 : Subsystem  TreatAsAtomicUnit=on
  cfblk11 : Delay  SampleTime=1
  cfblk12 : Delay  SampleTime=1
  cfblk3 : DiscreteFilter  SampleTime=1
  cfblk4 : Sin  TimeSource=Use external signal  SampleTime=0
  cfblk5 : Constant  Value=[-80148072.680011]  SampleTime=1
  cfblk6 : Subsystem
  cfblk7 : Subsystem
  cfblk8 : If  IfExpression=u1 >= 0  SampleTime=1
  cfblk9 : Subsystem  TreatAsAtomicUnit=on
  cfblk2 : Outport
  wires:
  cfblk10/1(cfblk2) -> cfblk4/1
  cfblk7/1(cfblk2) -> cfblk2/1
  cfblk10/2(cfblk11) -> cfblk6/1(cfblk1)
  cfblk5/1 -> cfblk10/1(cfblk1)
  cfblk7/2(cfblk14) -> cfblk3/1
  cfblk1/1 -> cfblk7/2(cfblk13)
  cfblk7/3(cfblk15) -> cfblk6/2(cfblk8), cfblk9/1(cfblk1)
  cfblk3/1 -> cfblk8/1
  cfblk9/1(cfblk2) -> cfblk6/3(cfblk9)
  cfblk9/2(cfblk9) -> cfblk10/3(cfblk10)
  cfblk8/1 -> cfblk9/Action
  cfblk8/2 -> cfblk10/Action
  cfblk6/1(cfblk2) -> cfblk11/1
  cfblk11/1 -> cfblk7/1(cfblk1)
  cfblk4/1 -> cfblk12/1
  cfblk12/1 -> cfblk10/2(cfblk9)

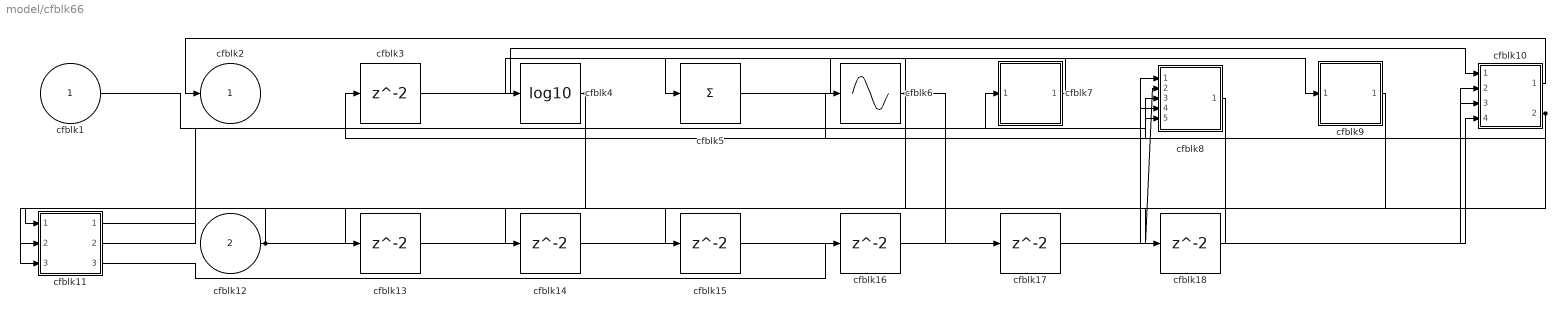
== system model/cfblk66 ==
  cfblk1 : Inport
  cfblk12 : Inport  Port=2
  cfblk10 : Subsystem
  cfblk11 : Subsystem
  cfblk{3,13..18} (7 alike) : Delay  SampleTime=1
  cfblk4 : Math  Operator=log10
  cfblk5 : Sum  Inputs=+
  cfblk6 : Sin  TimeSource=Use external signal  SampleTime=0
  cfblk7 : Subsystem
  cfblk8 : Subsystem
  cfblk9 : Subsystem
  cfblk2 : Outport
  wires:
  cfblk8/1(cfblk2) -> cfblk3/1
  cfblk3/1 -> cfblk10/1(cfblk1)
  cfblk12/1 -> cfblk8/2(cfblk8), cfblk11/1(cfblk1)
  cfblk7/1(cfblk2) -> cfblk5/1
  cfblk11/1(cfblk2) -> cfblk7/1(cfblk1)
  cfblk10/1(cfblk2) -> cfblk2/1
  cfblk5/1 -> cfblk9/1(cfblk1)
  cfblk4/1 -> cfblk11/2(cfblk11), cfblk13/1
  cfblk10/2(cfblk15) -> cfblk6/1, cfblk18/1
  cfblk1/1 -> cfblk8/3(cfblk9)
  cfblk6/1 -> cfblk4/1, cfblk11/3(cfblk12), cfblk17/1
  cfblk13/1 -> cfblk10/2(cfblk12)
  cfblk9/1(cfblk2) -> cfblk14/1
  cfblk14/1 -> cfblk8/1(cfblk1)
  cfblk11/2(cfblk13) -> cfblk15/1
  cfblk15/1 -> cfblk10/3(cfblk13)
  cfblk11/3(cfblk14) -> cfblk16/1
  cfblk16/1 -> cfblk10/4(cfblk14)
  cfblk17/1 -> cfblk8/4(cfblk10)
  cfblk18/1 -> cfblk8/5(cfblk11)

== system model/cfblk67 ==
  cfblk1 : Inport
  cfblk{10..13} (4 alike) : Delay  SampleTime=1
  cfblk3 : Bias  Bias=[-278903111.437649]  SaturateOnIntegerOverflow=off
  cfblk4 : ComplexToRealImag
  cfblk5 : ComplexToRealImag
  cfblk6 : Subsystem
  cfblk7 : Subsystem
  cfblk8 : Subsystem
  cfblk9 : Subsystem
  cfblk2 : Outport
  wires:
  cfblk6/1(cfblk2) -> cfblk7/1(cfblk1)
  cfblk6/2(cfblk10) -> cfblk7/2(cfblk8)
  cfblk9/1(cfblk2) -> cfblk4/1
  cfblk3/1 -> cfblk2/1
  cfblk8/1(cfblk2) -> cfblk3/1
  cfblk6/3(cfblk11) -> cfblk5/1
  cfblk4/1 -> cfblk8/1(cfblk1)
  cfblk9/2(cfblk15) -> cfblk8/2(cfblk10)
  cfblk1/1 -> cfblk9/3(cfblk14)
  cfblk8/3(cfblk13) -> cfblk6/1(cfblk1)
  cfblk5/2 -> cfblk7/3(cfblk9)
  cfblk8/4(cfblk14) -> cfblk6/2(cfblk8)
  cfblk4/2 -> cfblk7/4(cfblk10)
  cfblk8/2(cfblk12) -> cfblk10/1
  cfblk10/1 -> cfblk9/2(cfblk13)
  cfblk7/1(cfblk2) -> cfblk11/1
  cfblk11/1 -> cfblk8/3(cfblk11)
  cfblk7/2(cfblk11) -> cfblk12/1
  cfblk12/1 -> cfblk6/3(cfblk9)
  cfblk5/1 -> cfblk13/1
  cfblk13/1 -> cfblk9/1(cfblk1)
